simulink model "Linear_Transformation_Matrix"  (R2018a)
settings: Solver=VariableStepAuto  StartTime=0.0  StopTime=10.0  RelTol=1e-3
libraries: simulink_extras x3
settings Model: Creator=Ibrahim  LastModifiedBy=Ibrahim

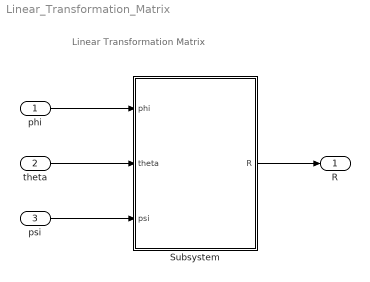
== system Linear_Transformation_Matrix ==
  note: Linear Transformation Matrix
  phi : Inport
  theta : Inport  Port=2
  psi : Inport  Port=3
  Subsystem : Subsystem
  R : Outport
  wires:
  phi/1 -> Subsystem/1(phi)
  theta/1 -> Subsystem/2(theta)
  psi/1 -> Subsystem/3(psi)
  Subsystem/1(R) -> R/1

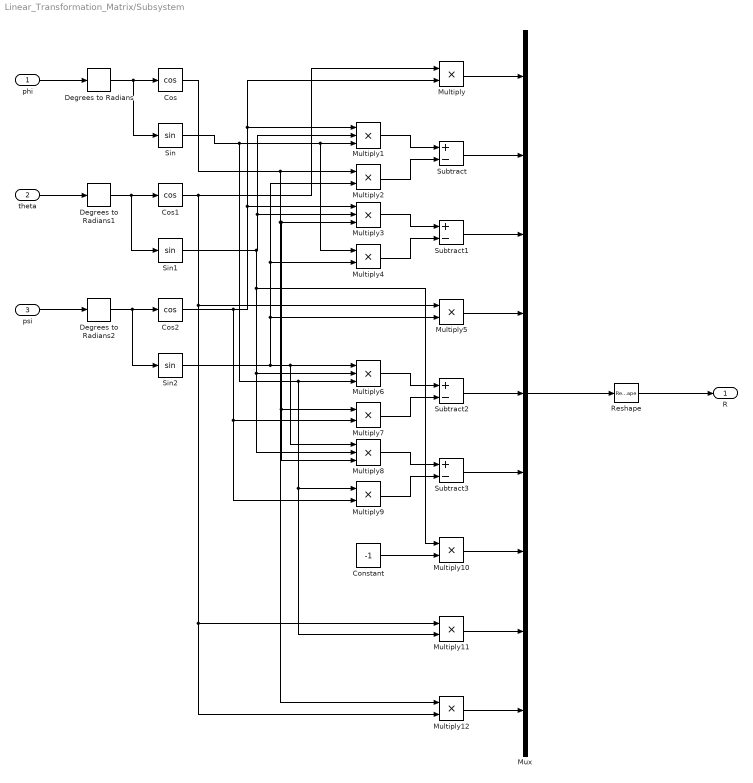
== system Linear_Transformation_Matrix/Subsystem ==
  phi : Inport
  theta : Inport  Port=2
  psi : Inport  Port=3
  Constant : Constant  Value=-1
  Cos : Trigonometry  Operator=cos
  Cos1 : Trigonometry  Operator=cos
  Cos2 : Trigonometry  Operator=cos
  Degrees to Radians : simulink_extras/Transformations/Degrees to Radians
  Degrees to Radians1 : simulink_extras/Transformations/Degrees to Radians
  Degrees to Radians2 : simulink_extras/Transformations/Degrees to Radians
  Multiply{,2,4..5,7,9..12} (9 alike) : Product
  Multiply{1,3,6,8} (4 alike) : Product  Inputs=3
  Mux : Mux  Inputs=9
  Reshape : Reshape  OutputDimensionality=Customize  OutputDimensions=[3,3]
  Sin : Trigonometry
  Sin1 : Trigonometry
  Sin2 : Trigonometry
  Subtract{,1..3} (4 alike) : Sum  Inputs=+-
  R : Outport
  wires:
  Constant/1 -> Multiply10/2
  Multiply11/1 -> Mux/8
  Multiply3/1 -> Subtract1/1
  Degrees to Radians2/1 -> Sin2/1, Cos2/1
  Sin2/1 -> Multiply8/1, Multiply6/1, Multiply5/2, Multiply4/2, Multiply2/2
  Mux/1 -> Reshape/1
  Multiply8/1 -> Subtract3/1
  Sin1/1 -> Multiply8/2, Multiply6/2, Multiply10/1, Multiply3/2, Multiply1/2
  Cos/1 -> Multiply8/3, Multiply7/1, Multiply3/3, Multiply12/1, Multiply2/1
  Cos1/1 -> Multiply5/1, Multiply12/2, Multiply11/1, Multiply/1
  Degrees to Radians/1 -> Cos/1, Sin/1
  phi/1 -> Degrees to Radians/1
  Degrees to Radians1/1 -> Sin1/1, Cos1/1
  Multiply/1 -> Mux/1
  Multiply10/1 -> Mux/7
  Reshape/1 -> R/1
  Sin/1 -> Multiply6/3, Multiply11/2, Multiply9/1, Multiply4/1, Multiply1/3
  Cos2/1 -> Multiply7/2, Multiply9/2, Multiply3/1, Multiply1/1, Multiply/2
  Multiply2/1 -> Subtract/2
  Multiply5/1 -> Mux/4
  Multiply1/1 -> Subtract/1
  Multiply12/1 -> Mux/9
  Subtract/1 -> Mux/2
  Subtract2/1 -> Mux/5
  theta/1 -> Degrees to Radians1/1
  Subtract3/1 -> Mux/6
  Subtract1/1 -> Mux/3
  Multiply7/1 -> Subtract2/2
  Multiply6/1 -> Subtract2/1
  Multiply4/1 -> Subtract1/2
  psi/1 -> Degrees to Radians2/1
  Multiply9/1 -> Subtract3/2
